simulink model "LowPass_Sim"  (R2022b)
settings: Solver=VariableStepAuto  StartTime=0.0  StopTime=10.0  RelTol=1e-3
values from neighbouring files (symbols this model uses):
  amplitude_input = 1    [LP_config.m]
  denGs = [1 wc]    [LP_config.m]
  denGz = cell2mat(Gz.Denominator)    [LP_config.m]
  numGs = [wc]    [LP_config.m]
  numGz = cell2mat(Gz.Numerator)    [LP_config.m]
  offset_input = 2.5    [LP_config.m]
  Ts = 1/f_sample    (= 0.0015873015873)    [LP_config.m]
  Tsim = 0.01*Ts    (= 1.5873015873e-05)    [LP_config.m]
  w_input = 2*pi*f_input    (= 3958.40674352)    [LP_config.m]
settings Model: Creator=mluser  LastModifiedBy=mluser
settings SFSimCC: SimCustomHeaderCode="#include \"LowPass.h\""  SimUserSources=LowPass.c  SimUserIncludeDirs=MATLAB Drive/Regulacion/Filtros/LowPass
settings RTWCC: RTWUseSimCustomCode=on  CustomHeaderCode="#include \"LowPass.h\""  CustomInclude=MATLAB Drive/Regulacion/Filtros/LowPass  CustomSource=LowPass.c

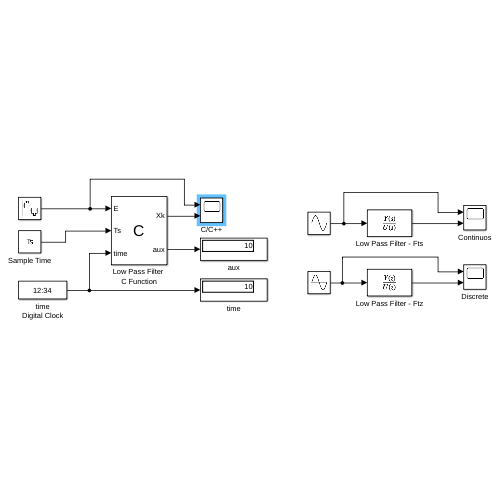
[thumbnail: Simulink's stored preview of the top-level diagram]
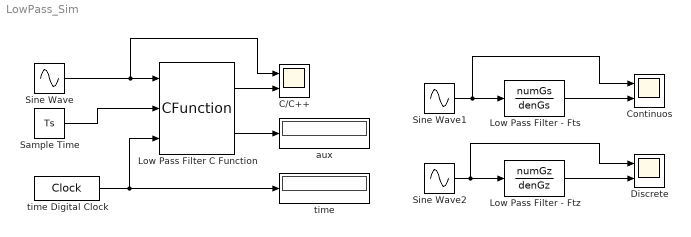
== system LowPass_Sim ==
  C/C++ : Scope  NumInputPorts=2
  Continuos : Scope  NumInputPorts=2
  Discrete : Scope  NumInputPorts=2
  Low Pass Filter C Function : CFunction  OutputCode=Xk=LowPass(E, Ts, time, &aux);
  Low Pass Filter - Fts : TransferFcn  Numerator=numGs  Denominator=denGs
  Low Pass Filter - Ftz : DiscreteTransferFcn  Numerator=numGz  Denominator=denGz  SampleTime=Ts
  Sample Time : Constant  Value=Ts
  Sine Wave : Sin  Amplitude=amplitude_input  Bias=offset_input  Frequency=w_input  SampleTime=Tsim
  Sine Wave1 : Sin  Amplitude=amplitude_input  Bias=offset_input  Frequency=w_input  SampleTime=0
  Sine Wave2 : Sin  Amplitude=amplitude_input  Bias=offset_input  Frequency=w_input  SampleTime=0
  aux : Display
  time : Display
  time Digital Clock : DigitalClock  SampleTime=Tsim
  wires:
  Low Pass Filter C Function/1 -> C/C++/2
  Sample Time/1 -> Low Pass Filter C Function/2
  time Digital Clock/1 -> time/1, Low Pass Filter C Function/3
  Sine Wave/1 -> Low Pass Filter C Function/1, C/C++/1
  Sine Wave1/1 -> Continuos/1, Low Pass Filter - Fts/1
  Low Pass Filter - Fts/1 -> Continuos/2
  Low Pass Filter - Ftz/1 -> Discrete/2
  Sine Wave2/1 -> Discrete/1, Low Pass Filter - Ftz/1
  Low Pass Filter C Function/2 -> aux/1
